simulink model "ex1b"  (R2015a)
settings: Solver=ode45  StartTime=0.0  StopTime=10  RelTol=1e-3
values from neighbouring files (symbols this model uses):
  D = [1 2 4]    [ex1.m]
  k = 1    [ex1.m]
  m = 1    [ex1.m]
settings Model: Creator=martinspedro  LastModifiedBy=martinspedro

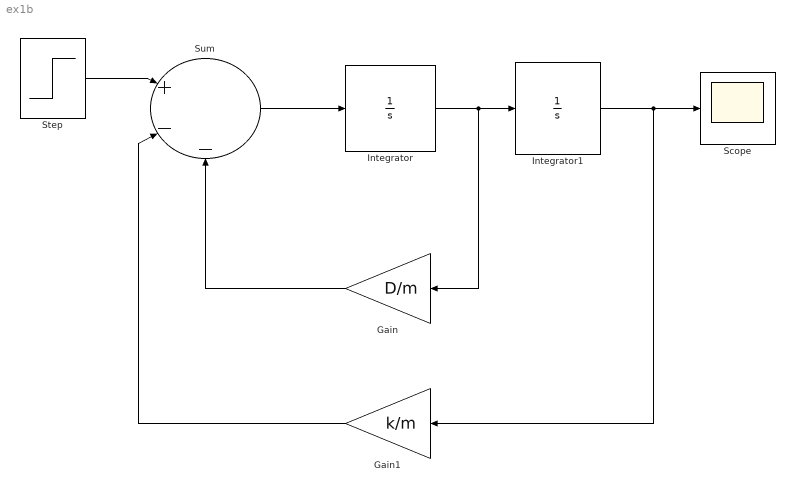
== system ex1b ==
  Gain : Gain  Gain=D/m
  Gain1 : Gain  Gain=k/m
  Integrator : Integrator
  Integrator1 : Integrator
  Scope : Scope
      settings: ShowLegends=on
  Step : Step  Time=0  SampleTime=0
  Sum : Sum  Inputs=|+--
  wires:
  Sum/1 -> Integrator/1
  Integrator/1 -> Gain/1, Integrator1/1
  Integrator1/1 -> Gain1/1, Scope/1
  Gain1/1 -> Sum/2
  Gain/1 -> Sum/3
  Step/1 -> Sum/1
